simulink model "Lab_1"  (R2017b)
settings: Solver=ode45  StartTime=0.0  StopTime=50  RelTol=1e-3
values from neighbouring files (symbols this model uses):
  I_1 = 0.109    [main.m]
  I_2 = 0.0504    [main.m]
  I_3 = 0.0504    [main.m]
settings Model: Creator=fcuzzocrea  LastModifiedBy=fcuzzocrea

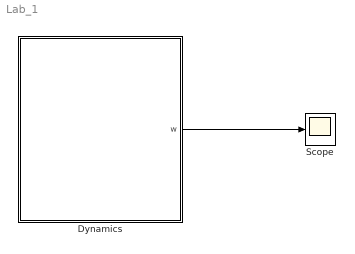
== system Lab_1 ==
  "Dynamics " : Subsystem
  Scope : Scope
  wires:
  "Dynamics "/1(w) -> Scope/1

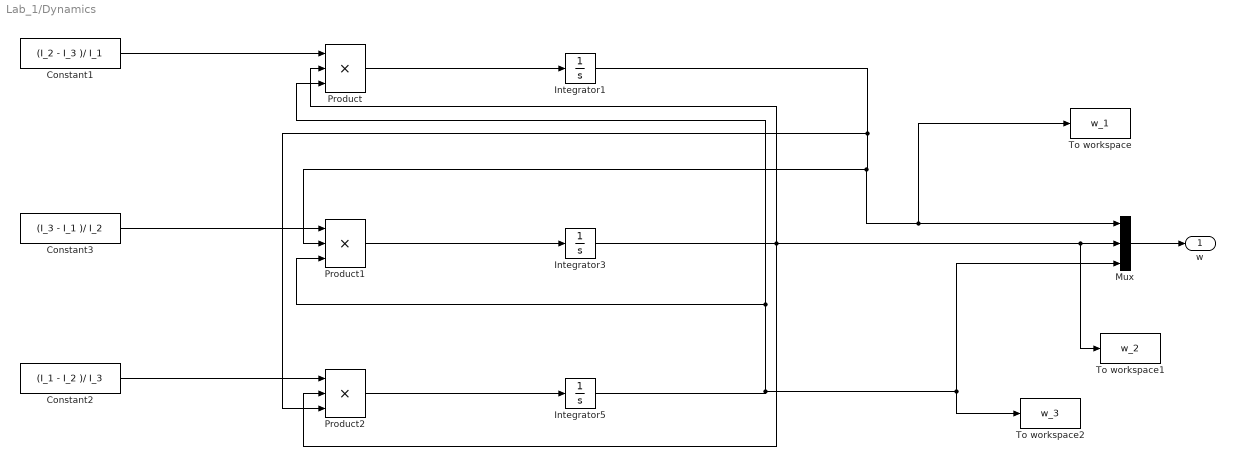
== system Lab_1/Dynamics  ==
  Constant1 : Constant  Value=(I_2 - I_3 )/ I_1
  Constant2 : Constant  Value=(I_1 - I_2 )/ I_3
  Constant3 : Constant  Value=(I_3 - I_1 )/ I_2
  Integrator1 : Integrator
  Integrator3 : Integrator  InitialCondition=0.45
  Integrator5 : Integrator  InitialCondition=0.26
  Mux : Mux  Inputs=3
  Product : Product  Inputs=3
  Product1 : Product  Inputs=3
  Product2 : Product  Inputs=3
  To workspace : ToWorkspace  VariableName=w_1  SampleTime=-1
  To workspace1 : ToWorkspace  VariableName=w_2  SampleTime=-1
  To workspace2 : ToWorkspace  VariableName=w_3  SampleTime=-1
  w : Outport
  wires:
  Integrator3/1 -> To workspace1/1, Mux/2, Product2/2, Product/2
  Integrator5/1 -> Mux/3, To workspace2/1, Product/3, Product1/3
  Product1/1 -> Integrator3/1
  Product2/1 -> Integrator5/1
  Constant1/1 -> Product/1
  Constant3/1 -> Product1/1
  Constant2/1 -> Product2/1
  Integrator1/1 -> Product2/3, To workspace/1, Mux/1, Product1/2
  Product/1 -> Integrator1/1
  Mux/1 -> w/1
